simulink model "PSFq"  (R2014a)
settings: Solver=ode45  StartTime=0.0  StopTime=700  RelTol=1e-3
values from neighbouring files (symbols this model uses):
  d = Pd.iodelay    [PSFEsta.m]
  Ts = 0.4    [PSFEsta.m]
libraries: cstblocks x5
settings Model: Creator=Sergio  LastModifiedBy=Sergio

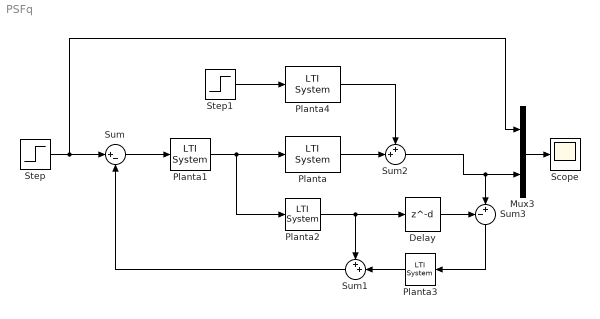
== system PSFq ==
  Delay : Delay  DelayLength=d  SampleTime=Ts
  Mux3 : Mux  Inputs=2
  Planta : cstblocks/LTI System  sys=Pdn  IC=[36]
  Planta1 : cstblocks/LTI System  sys=Cd  IC=[36]
  Planta2 : cstblocks/LTI System  sys=Gnd  IC=[36]
  Planta3 : cstblocks/LTI System  sys=Fr  IC=[36]
  Planta4 : cstblocks/LTI System  sys=Pq  IC=[36]
  Scope : Scope
  Step : Step  Time=0  SampleTime=Ts
  Step1 : Step  Time=300  SampleTime=Ts
  Sum : Sum  Inputs=|+-  SampleTime=Ts
  Sum1 : Sum  Inputs=++|  SampleTime=Ts
  Sum2 : Sum  Inputs=++|  SampleTime=Ts
  Sum3 : Sum  Inputs=-+|  SampleTime=Ts
  wires:
  Step/1 -> Mux3/1, Sum/1
  Sum/1 -> Planta1/1
  Planta1/1 -> Planta2/1, Planta/1
  Planta3/1 -> Sum1/2
  Planta/1 -> Sum2/2
  Sum2/1 -> Mux3/2, Sum3/2
  Sum1/1 -> Sum/2
  Planta4/1 -> Sum2/1
  Step1/1 -> Planta4/1
  Mux3/1 -> Scope/1
  Planta2/1 -> Sum1/1, Delay/1
  Delay/1 -> Sum3/1
  Sum3/1 -> Planta3/1
